simulink model "Appl_PaAdjustModel"  (R2018b)
settings: configuration reference "CodeConfig_10_ms" (kept outside this file)
undefined symbols (not defined in the file): CAL_HightMotorRunInterval_100ms, CAL_MotorDiffToStart_100ms, CAL_MotorStopTime_50ms, D_Relay_DownBackFault, D_Relay_UpFrontFault, D_ToleranceDistance, enSeatMoveCmd, FALSE, TRUE
libraries: DareLib x84, simulink x2
(part 1 of 3)
settings Model: Creator=Administrator  LastModifiedBy=Administrator
settings ConfigSetRef: SourceLocation=Base Workspace

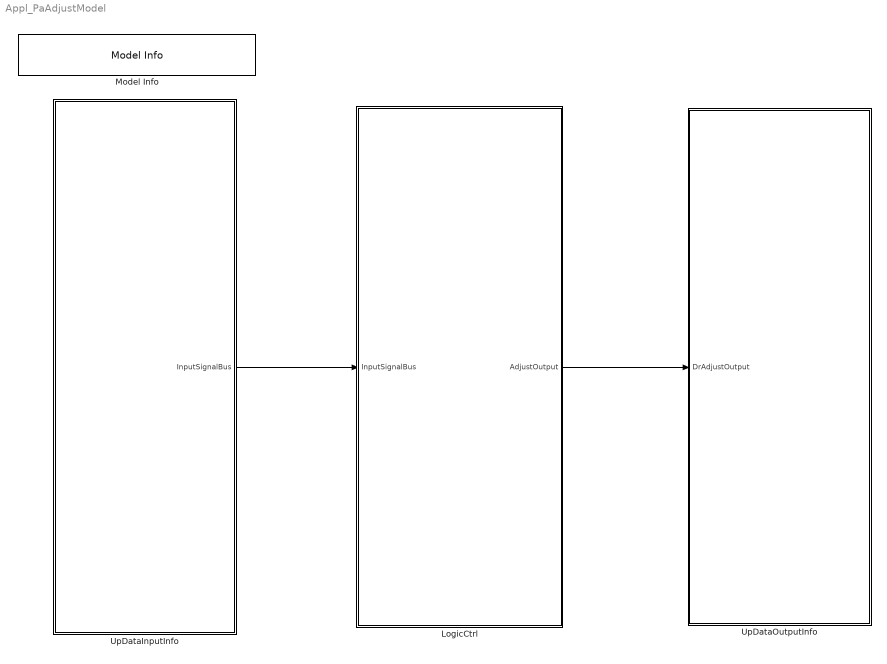
== system Appl_PaAdjustModel ==
  LogicCtrl : Subsystem  Priority=2  TreatAsAtomicUnit=on
      settings: RTWSystemCode=Nonreusable function  RTWFcnNameOpts=Use subsystem name
  Model Info : simulink/Model-Wide Utilities/Model Info  Frame=on  DisplayStringWithTags=Version：%<ModelVersion>  HorizontalTextAlignment=Center  LeftAlignmentValue=0.5
  UpDataInputInfo : Subsystem  Priority=1  TreatAsAtomicUnit=on
      settings: RTWSystemCode=Nonreusable function  RTWFcnNameOpts=Use subsystem name
  UpDataOutputInfo : Subsystem  Priority=3  TreatAsAtomicUnit=on
      settings: RTWSystemCode=Nonreusable function  RTWFcnNameOpts=Use subsystem name
  wires:
  UpDataInputInfo/1(InputSignalBus) -> LogicCtrl/1(InputSignalBus)
  LogicCtrl/1(AdjustOutput) -> UpDataOutputInfo/1(DrAdjustOutput)

== system Appl_PaAdjustModel/LogicCtrl ==
  InputSignalBus : Inport
  LocalAdjustCtrl : Subsystem  Description=调节逻辑处理
      settings: AttributesFormatString=%<Description>
  AdjustOutput : Outport
  wires:
  InputSignalBus/1 -> LocalAdjustCtrl/1(RteInputBus)  "RteInputBus"
  LocalAdjustCtrl/1(LocalAdjustCtrlOut) -> AdjustOutput/1

== system Appl_PaAdjustModel/UpDataInputInfo ==
  InputSignalProcess : Subsystem  Description=数据处理
      settings: AttributesFormatString=%<Description>  RTWSystemCode=Nonreusable function  RTWFcnNameOpts=Use subsystem name
  RTE : Subsystem  Description=接口自动生成  TreatAsAtomicUnit=on
      settings: AttributesFormatString=%<Description>  RTWSystemCode=Nonreusable function  RTWFcnNameOpts=Use subsystem name
  InputSignalBus : Outport
  wires:
  InputSignalProcess/1(InputSignalBus) -> InputSignalBus/1
  RTE/1(RTE_Signal) -> InputSignalProcess/1(Rte_SignalBus)

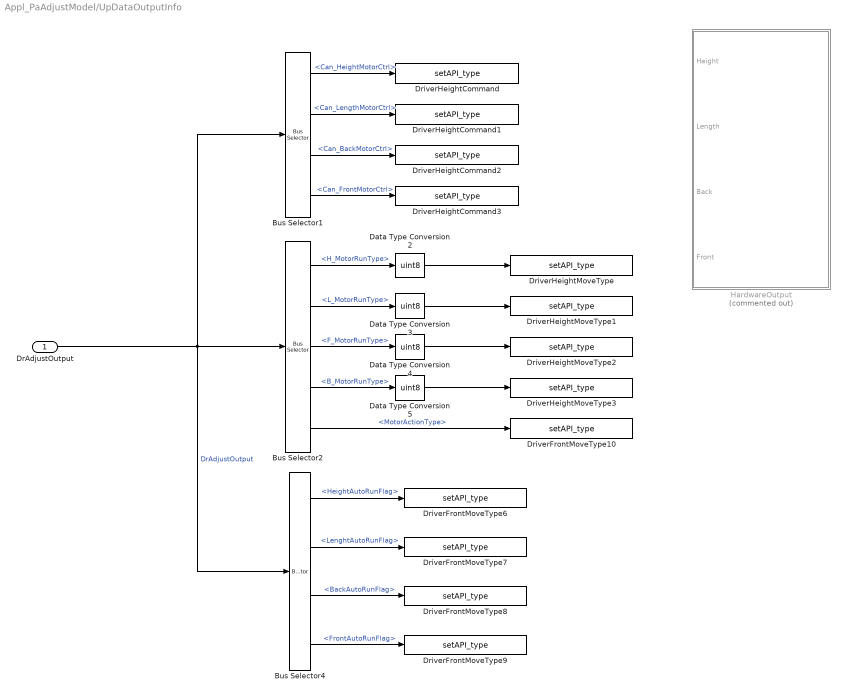
== system Appl_PaAdjustModel/UpDataOutputInfo ==
  DrAdjustOutput : Inport
  Bus Selector1 : BusSelector  OutputSignals=MotorCtrl.Can_HeightMotorCtrl,MotorCtrl.Can_LengthMotorCtrl,MotorCtrl.Can_BackMotorCtrl,MotorCtrl.Can_FrontMotorCtrl
  Bus Selector2 : BusSelector  OutputSignals=MotorRunType.H_MotorRunType,MotorRunType.L_MotorRunType,MotorRunType.F_MotorRunType,MotorRunType.B_MotorRunType,MotorReq.MotorActionType
  Bus Selector4 : BusSelector  OutputSignals=AutoRunFlag.HeightAutoRunFlag,AutoRunFlag.LenghtAutoRunFlag,AutoRunFlag.BackAutoRunFlag,AutoRunFlag.FrontAutoRunFlag
  Data Type Conversion{2..5} (4 alike) : DataTypeConversion  OutDataTypeStr=uint8
  DriverFrontMoveType10 : DareLib/Dare/setAPI_type  g_funcname=Rte_SetVfb_PaMoveType  g_param=""  g_type=uint8  g_enum=enSeatMotorRunTye  g_size=-1
      settings: AttributesFormatString=%<g_funcname>  SourceProductName=Dare Library
  DriverFrontMoveType6 : DareLib/Dare/setAPI_type  g_funcname=Rte_SetVfb_PaHeightAutoRunFlag  g_param=""  g_type=uint8  g_enum=enSeatAutoRunSts  g_size=-1
      settings: AttributesFormatString=%<g_funcname>  SourceProductName=Dare Library
  DriverFrontMoveType7 : DareLib/Dare/setAPI_type  g_funcname=Rte_SetVfb_PaLengthAutoRunFlag  g_param=""  g_type=uint8  g_enum=enSeatAutoRunSts  g_size=-1
      settings: AttributesFormatString=%<g_funcname>  SourceProductName=Dare Library
  DriverFrontMoveType8 : DareLib/Dare/setAPI_type  g_funcname=Rte_SetVfb_PaBackAutoRunFlag  g_param=""  g_type=uint8  g_enum=enSeatAutoRunSts  g_size=-1
      settings: AttributesFormatString=%<g_funcname>  SourceProductName=Dare Library
  DriverFrontMoveType9 : DareLib/Dare/setAPI_type  g_funcname=Rte_SetVfb_PaFrontAutoRunFlag  g_param=""  g_type=uint8  g_enum=enSeatAutoRunSts  g_size=-1
      settings: AttributesFormatString=%<g_funcname>  SourceProductName=Dare Library
  DriverHeightCommand : DareLib/Dare/setAPI_type  g_funcname=Rte_SetVfb_PaHeightMotorCmd  g_param=""  g_type=uint8  g_size=-1
      settings: AttributesFormatString=%<g_funcname>  SourceProductName=Dare Library
  DriverHeightCommand1 : DareLib/Dare/setAPI_type  g_funcname=Rte_SetVfb_PaLengthMotorCmd  g_param=""  g_type=uint8  g_size=-1
      settings: AttributesFormatString=%<g_funcname>  SourceProductName=Dare Library
  DriverHeightCommand2 : DareLib/Dare/setAPI_type  g_funcname=Rte_SetVfb_PaBackMotorCmd  g_param=""  g_type=uint8  g_size=-1
      settings: AttributesFormatString=%<g_funcname>  SourceProductName=Dare Library
  DriverHeightCommand3 : DareLib/Dare/setAPI_type  g_funcname=Rte_SetVfb_PaFrontMotorCmd  g_param=""  g_type=uint8  g_size=-1
      settings: AttributesFormatString=%<g_funcname>  SourceProductName=Dare Library
  DriverHeightMoveType : DareLib/Dare/setAPI_type  g_funcname=Rte_SetVfb_PaHeightMotorReason  g_param=""  g_type=uint8  g_size=-1
      settings: AttributesFormatString=%<g_funcname>  SourceProductName=Dare Library
  DriverHeightMoveType1 : DareLib/Dare/setAPI_type  g_funcname=Rte_SetVfb_PaLengthMotorReason  g_param=""  g_type=uint8  g_size=-1
      settings: AttributesFormatString=%<g_funcname>  SourceProductName=Dare Library
  DriverHeightMoveType2 : DareLib/Dare/setAPI_type  g_funcname=Rte_SetVfb_PaBackMotorReason  g_param=""  g_type=uint8  g_size=-1
      settings: AttributesFormatString=%<g_funcname>  SourceProductName=Dare Library
  DriverHeightMoveType3 : DareLib/Dare/setAPI_type  g_funcname=Rte_SetVfb_PaFrontMotorReason  g_param=""  g_type=uint8  g_size=-1
      settings: AttributesFormatString=%<g_funcname>  SourceProductName=Dare Library
  HardwareOutput : Subsystem  Commented=on
  wires:
  DrAdjustOutput/1 -> Bus Selector4/1, Bus Selector1/1, Bus Selector2/1  "DrAdjustOutput"
  Data Type Conversion2/1 -> DriverHeightMoveType/1
  Data Type Conversion3/1 -> DriverHeightMoveType1/1
  Data Type Conversion4/1 -> DriverHeightMoveType2/1
  Data Type Conversion5/1 -> DriverHeightMoveType3/1
  Bus Selector1/1 -> DriverHeightCommand/1  "<Can_HeightMotorCtrl>"
  Bus Selector1/2 -> DriverHeightCommand1/1  "<Can_LengthMotorCtrl>"
  Bus Selector1/3 -> DriverHeightCommand2/1  "<Can_BackMotorCtrl>"
  Bus Selector1/4 -> DriverHeightCommand3/1  "<Can_FrontMotorCtrl>"
  Bus Selector2/1 -> Data Type Conversion2/1  "<H_MotorRunType>"
  Bus Selector2/2 -> Data Type Conversion3/1  "<L_MotorRunType>"
  Bus Selector2/3 -> Data Type Conversion4/1  "<F_MotorRunType>"
  Bus Selector2/4 -> Data Type Conversion5/1  "<B_MotorRunType>"
  Bus Selector2/5 -> DriverFrontMoveType10/1  "<MotorActionType>"
  Bus Selector4/2 -> DriverFrontMoveType7/1  "<LenghtAutoRunFlag>"
  Bus Selector4/1 -> DriverFrontMoveType6/1  "<HeightAutoRunFlag>"
  Bus Selector4/3 -> DriverFrontMoveType8/1  "<BackAutoRunFlag>"
  Bus Selector4/4 -> DriverFrontMoveType9/1  "<FrontAutoRunFlag>"

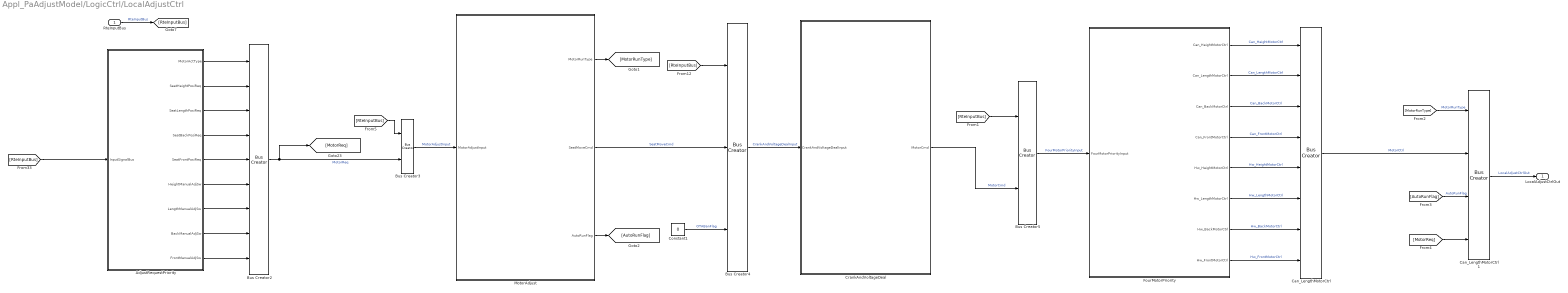
== system Appl_PaAdjustModel/LogicCtrl/LocalAdjustCtrl ==
  RteInputBus : Inport
  AdjustRequestPriority : Subsystem  Description=电机运动请求优先级处理
      settings: AttributesFormatString=%<Description>
      mask Display: image('优先级.png');
  Bus Creator2 : BusCreator  Inputs=9
  Bus Creator3 : BusCreator  Inputs=2
  Bus Creator4 : BusCreator  Inputs=3
  Bus Creator5 : BusCreator  Inputs=2
  Can_LengthMotorCtrl : BusCreator  Inputs=8
  Can_LengthMotorCtrl1 : BusCreator  Inputs=4
  Constant1 : Constant  Value=0
  CrankAndVoltageDeal : Subsystem  Description=CRANK卸荷和电压限制处理
      settings: AttributesFormatString=%<Description>
      mask Display: image('卸荷.png');
  FourMotorPriority : Subsystem  Description=四向调节电机运动优先级
      settings: AttributesFormatString=%<Description>
      mask Display: image('电机优先级.png');
  MotorAdjust : Subsystem  Description=四向电机调节
      settings: AttributesFormatString=%<Description>
      mask Display: image('电机调节.png');
  LocalAdjustCtrlOut : Outport
  wires:
  MotorAdjust/3(AutoRunFlag) -> [AutoRunFlag]
  [RteInputBus] -> Bus Creator4/1
  RteInputBus/1 -> [RteInputBus]  "RteInputBus"
  Bus Creator2/1 -> [MotorReq], Bus Creator3/2  "MotorReq"
  [RteInputBus] -> Bus Creator3/1
  Bus Creator3/1 -> MotorAdjust/1(MotorAdjustInput)  "MotorAdjustInput"
  Constant1/1 -> Bus Creator4/3  "OTABanFlag"
  MotorAdjust/2(SeatMoveCmd) -> Bus Creator4/2  "SeatMoveCmd"
  Bus Creator4/1 -> CrankAndVoltageDeal/1(CrankAndVoltageDealInput)  "CrankAndVoltageDealInput"
  CrankAndVoltageDeal/1(MotorCmd) -> Bus Creator5/2  "MotorCmd"
  [RteInputBus] -> Bus Creator5/1
  Bus Creator5/1 -> FourMotorPriority/1(FourMotorPriorityInput)  "FourMotorPriorityInput"
  MotorAdjust/1(MotorRunType) -> [MotorRunType]
  [MotorRunType] -> Can_LengthMotorCtrl1/1  "MotorRunType"
  [AutoRunFlag] -> Can_LengthMotorCtrl1/3  "AutoRunFlag"
  Can_LengthMotorCtrl/1 -> Can_LengthMotorCtrl1/2  "MotorCtrl"
  Can_LengthMotorCtrl1/1 -> LocalAdjustCtrlOut/1  "LocalAdjustCtrlOut"
  [MotorReq] -> Can_LengthMotorCtrl1/4
  AdjustRequestPriority/1(MotorActType) -> Bus Creator2/1
  AdjustRequestPriority/2(SeatHeightPosiReq) -> Bus Creator2/2
  AdjustRequestPriority/3(SeatLengthPosiReq) -> Bus Creator2/3
  AdjustRequestPriority/4(SeatBackPosiReq) -> Bus Creator2/4
  AdjustRequestPriority/5(SeatFrontPosiReq) -> Bus Creator2/5
  AdjustRequestPriority/6(HeightManualAdjSw) -> Bus Creator2/6
  AdjustRequestPriority/7(LengthManualAdjSw) -> Bus Creator2/7
  AdjustRequestPriority/8(BackManualAdjSw) -> Bus Creator2/8
  AdjustRequestPriority/9(FrontManualAdjSw) -> Bus Creator2/9
  FourMotorPriority/1(Can_HeightMotorCtrl) -> Can_LengthMotorCtrl/1  "Can_HeightMotorCtrl"
  FourMotorPriority/2(Can_LengthMotorCtrl) -> Can_LengthMotorCtrl/2  "Can_LengthMotorCtrl"
  FourMotorPriority/3(Can_BackMotorCtrl) -> Can_LengthMotorCtrl/3  "Can_BackMotorCtrl"
  FourMotorPriority/4(Can_FrontMotorCtrl) -> Can_LengthMotorCtrl/4  "Can_FrontMotorCtrl"
  FourMotorPriority/5(Hw_HeightMotorCtrl) -> Can_LengthMotorCtrl/5  "Hw_HeightMotorCtrl"
  FourMotorPriority/6(Hw_LengthMotorCtrl) -> Can_LengthMotorCtrl/6  "Hw_LengthMotorCtrl"
  FourMotorPriority/7(Hw_BackMotorCtrl) -> Can_LengthMotorCtrl/7  "Hw_BackMotorCtrl"
  FourMotorPriority/8(Hw_FrontMotorCtrl) -> Can_LengthMotorCtrl/8  "Hw_FrontMotorCtrl"
  [RteInputBus] -> AdjustRequestPriority/1(InputSignalBus)

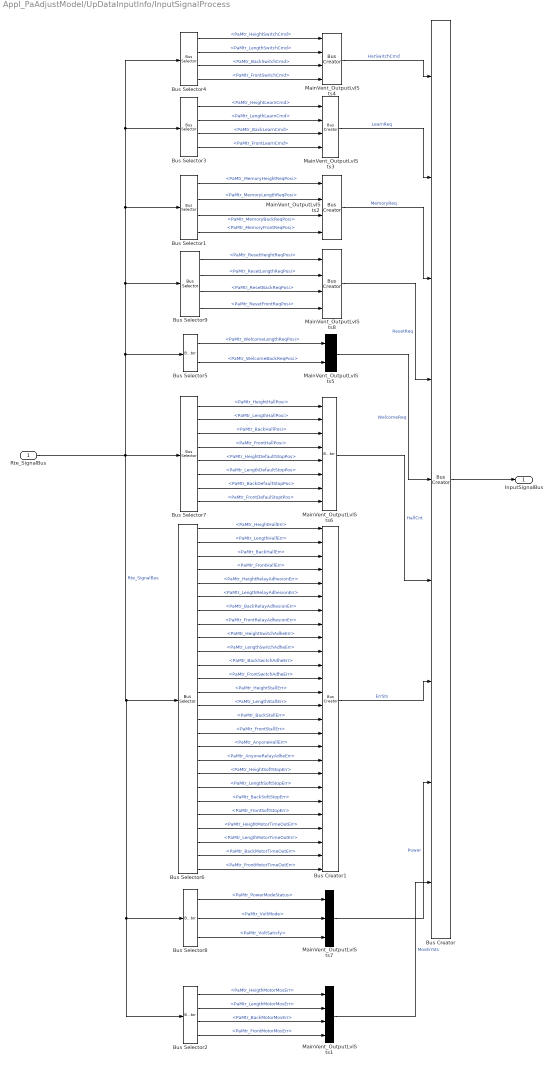
== system Appl_PaAdjustModel/UpDataInputInfo/InputSignalProcess ==
  Rte_SignalBus : Inport
  Bus Creator : BusCreator  Inputs=9
  Bus Creator1 : BusCreator  Inputs=26
  Bus Selector1 : BusSelector  OutputSignals=PaMtr_MemoryHeightReqPosi,PaMtr_MemoryLengthReqPosi,PaMtr_MemoryBackReqPosi,PaMtr_MemoryFrontReqPosi
  Bus Selector2 : BusSelector  OutputSignals=PaMtr_HeigthMotorMosErr,PaMtr_LengthMotorMosErr,PaMtr_BackMotorMosErr,PaMtr_FrontMotorMosErr
  Bus Selector3 : BusSelector  OutputSignals=PaMtr_HeightLearnCmd,PaMtr_LengthLearnCmd,PaMtr_BackLearnCmd,PaMtr_FrontLearnCmd
  Bus Selector4 : BusSelector  OutputSignals=PaMtr_HeightSwitchCmd,PaMtr_LengthSwitchCmd,PaMtr_BackSwitchCmd,PaMtr_FrontSwitchCmd
  Bus Selector5 : BusSelector  OutputSignals=PaMtr_WelcomeLengthReqPosi,PaMtr_WelcomeBackReqPosi
  Bus Selector6 : BusSelector  OutputSignals=PaMtr_HeightHallErr,PaMtr_LengthHallErr,PaMtr_BackHallErr,PaMtr_FrontHallErr,PaMtr_HeightRelayAdhesionErr,PaMtr_LengthRelayAdhesionErr,PaMtr_BackRelayAdhesionErr,PaMtr_FrontRelayAdhesionErr,PaMtr_HeightSwitchAdheErr,PaMtr_LengthSwitchAdheErr,PaMtr_BackSwitchAdheErr,PaMtr_FrontSwitchAdheErr,PaMtr_HeightStallErr,PaMtr_LengthStallErr,PaMtr_BackStallErr,PaMtr_FrontStallErr,PaMtr_AnyoneHallErr,PaMtr_AnyoneRelayAdheErr,PaMtr_HeightSoftStopErr,PaMtr_LengthSoftStopErr,PaMtr_BackSoftStopErr,PaMtr_FrontSoftStopErr,PaMtr_HeightMotorTimeOutErr,PaMtr_LengthMotorTimeOutErr,PaMtr_BackMotorTimeOutErr,PaMtr_FrontMotorTimeOutErr
  Bus Selector7 : BusSelector  OutputSignals=PaMtr_HeightHallPosi,PaMtr_LengthHallPosi,PaMtr_BackHallPosi,PaMtr_FrontHallPosi,PaMtr_HeightDefaultStopPos,PaMtr_LengthDefaultStopPos,PaMtr_BackDefaultStopPos,PaMtr_FrontDefaulStoptPos
  Bus Selector8 : BusSelector  OutputSignals=PaMtr_PowerModeStatus,PaMtr_VoltMode,PaMtr_VoltSatisfy
  Bus Selector9 : BusSelector  OutputSignals=PaMtr_ResetHeightReqPosi,PaMtr_ResetLengthReqPosi,PaMtr_ResetBackReqPosi,PaMtr_ResetFrontReqPosi
  MainVent_OutputLvlSts{1..4,8} (5 alike) : BusCreator  Inputs=4
  MainVent_OutputLvlSts5 : BusCreator  Inputs=2
  MainVent_OutputLvlSts6 : BusCreator  Inputs=8
  MainVent_OutputLvlSts7 : BusCreator  Inputs=3
  InputSignalBus : Outport
  wires:
  Bus Creator/1 -> InputSignalBus/1
  Bus Selector4/1 -> MainVent_OutputLvlSts4/1  "<PaMtr_HeightSwitchCmd>"
  Bus Selector4/2 -> MainVent_OutputLvlSts4/2  "<PaMtr_LengthSwitchCmd>"
  Bus Selector4/3 -> MainVent_OutputLvlSts4/3  "<PaMtr_BackSwitchCmd>"
  Bus Selector4/4 -> MainVent_OutputLvlSts4/4  "<PaMtr_FrontSwitchCmd>"
  Bus Selector7/1 -> MainVent_OutputLvlSts6/1  "<PaMtr_HeightHallPosi>"
  Bus Selector7/2 -> MainVent_OutputLvlSts6/2  "<PaMtr_LengthHallPosi>"
  Bus Selector7/3 -> MainVent_OutputLvlSts6/3  "<PaMtr_BackHallPosi>"
  Bus Selector7/4 -> MainVent_OutputLvlSts6/4  "<PaMtr_FrontHallPosi>"
  Bus Selector7/5 -> MainVent_OutputLvlSts6/5  "<PaMtr_HeightDefaultStopPos>"
  Bus Selector7/6 -> MainVent_OutputLvlSts6/6  "<PaMtr_LengthDefaultStopPos>"
  Bus Selector7/7 -> MainVent_OutputLvlSts6/7  "<PaMtr_BackDefaultStopPos>"
  Bus Selector8/2 -> MainVent_OutputLvlSts7/2  "<PaMtr_VoltMode>"
  Bus Selector8/1 -> MainVent_OutputLvlSts7/1  "<PaMtr_PowerModeStatus>"
  Bus Selector8/3 -> MainVent_OutputLvlSts7/3  "<PaMtr_VoltSatisfy>"
  MainVent_OutputLvlSts7/1 -> Bus Creator/8  "Power"
  MainVent_OutputLvlSts4/1 -> Bus Creator/1  "HarSwitchCmd"
  MainVent_OutputLvlSts2/1 -> Bus Creator/3  "MemoryReq"
  Bus Creator1/1 -> Bus Creator/7  "ErrSts"
  MainVent_OutputLvlSts5/1 -> Bus Creator/5  "WelcomeReq"
  MainVent_OutputLvlSts6/1 -> Bus Creator/6  "HallCnt"
  Bus Selector6/1 -> Bus Creator1/1  "<PaMtr_HeightHallErr>"
  Bus Selector6/2 -> Bus Creator1/2  "<PaMtr_LengthHallErr>"
  Bus Selector6/3 -> Bus Creator1/3  "<PaMtr_BackHallErr>"
  Bus Selector6/4 -> Bus Creator1/4  "<PaMtr_FrontHallErr>"
  Bus Selector6/5 -> Bus Creator1/5  "<PaMtr_HeightRelayAdhesionErr>"
  Bus Selector6/6 -> Bus Creator1/6  "<PaMtr_LengthRelayAdhesionErr>"
  Bus Selector6/7 -> Bus Creator1/7  "<PaMtr_BackRelayAdhesionErr>"
  Bus Selector6/8 -> Bus Creator1/8  "<PaMtr_FrontRelayAdhesionErr>"
  Bus Selector6/9 -> Bus Creator1/9  "<PaMtr_HeightSwitchAdheErr>"
  Bus Selector6/10 -> Bus Creator1/10  "<PaMtr_LengthSwitchAdheErr>"
  Bus Selector6/11 -> Bus Creator1/11  "<PaMtr_BackSwitchAdheErr>"
  Bus Selector6/12 -> Bus Creator1/12  "<PaMtr_FrontSwitchAdheErr>"
  Bus Selector6/13 -> Bus Creator1/13  "<PaMtr_HeightStallErr>"
  Bus Selector6/14 -> Bus Creator1/14  "<PaMtr_LengthStallErr>"
  Bus Selector6/15 -> Bus Creator1/15  "<PaMtr_BackStallErr>"
  Bus Selector6/16 -> Bus Creator1/16  "<PaMtr_FrontStallErr>"
  Bus Selector6/17 -> Bus Creator1/17  "<PaMtr_AnyoneHallErr>"
  Bus Selector6/18 -> Bus Creator1/18  "<PaMtr_AnyoneRelayAdheErr>"
  Bus Selector6/19 -> Bus Creator1/19  "<PaMtr_HeightSoftStopErr>"
  Bus Selector6/20 -> Bus Creator1/20  "<PaMtr_LengthSoftStopErr>"
  Bus Selector6/21 -> Bus Creator1/21  "<PaMtr_BackSoftStopErr>"
  Bus Selector6/22 -> Bus Creator1/22  "<PaMtr_FrontSoftStopErr>"
  Bus Selector6/23 -> Bus Creator1/23  "<PaMtr_HeightMotorTimeOutErr>"
  Bus Selector6/24 -> Bus Creator1/24  "<PaMtr_LengthMotorTimeOutErr>"
  Bus Selector6/25 -> Bus Creator1/25  "<PaMtr_BackMotorTimeOutErr>"
  Bus Selector6/26 -> Bus Creator1/26  "<PaMtr_FrontMotorTimeOutErr>"
  Bus Selector1/3 -> MainVent_OutputLvlSts2/3  "<PaMtr_MemoryBackReqPosi>"
  Bus Selector1/2 -> MainVent_OutputLvlSts2/2  "<PaMtr_MemoryLengthReqPosi>"
  Bus Selector1/4 -> MainVent_OutputLvlSts2/4  "<PaMtr_MemoryFrontReqPosi>"
  Bus Selector1/1 -> MainVent_OutputLvlSts2/1  "<PaMtr_MemoryHeightReqPosi>"
  Bus Selector5/1 -> MainVent_OutputLvlSts5/1  "<PaMtr_WelcomeLengthReqPosi>"
  Bus Selector5/2 -> MainVent_OutputLvlSts5/2  "<PaMtr_WelcomeBackReqPosi>"
  Bus Selector7/8 -> MainVent_OutputLvlSts6/8  "<PaMtr_FrontDefaulStoptPos>"
  Bus Selector3/1 -> MainVent_OutputLvlSts3/1  "<PaMtr_HeightLearnCmd>"
  Bus Selector3/2 -> MainVent_OutputLvlSts3/2  "<PaMtr_LengthLearnCmd>"
  Bus Selector3/3 -> MainVent_OutputLvlSts3/3  "<PaMtr_BackLearnCmd>"
  Bus Selector3/4 -> MainVent_OutputLvlSts3/4  "<PaMtr_FrontLearnCmd>"
  MainVent_OutputLvlSts3/1 -> Bus Creator/2  "LearnReq"
  Bus Selector9/1 -> MainVent_OutputLvlSts8/1  "<PaMtr_ResetHeightReqPosi>"
  Bus Selector9/2 -> MainVent_OutputLvlSts8/2  "<PaMtr_ResetLengthReqPosi>"
  Bus Selector9/4 -> MainVent_OutputLvlSts8/4  "<PaMtr_ResetFrontReqPosi>"
  Bus Selector9/3 -> MainVent_OutputLvlSts8/3  "<PaMtr_ResetBackReqPosi>"
  MainVent_OutputLvlSts8/1 -> Bus Creator/4  "ResetReq"
  MainVent_OutputLvlSts1/1 -> Bus Creator/9  "MosErrSts"
  Bus Selector2/3 -> MainVent_OutputLvlSts1/3  "<PaMtr_BackMotorMosErr>"
  Bus Selector2/2 -> MainVent_OutputLvlSts1/2  "<PaMtr_LengthMotorMosErr>"
  Rte_SignalBus/1 -> Bus Selector2/1, Bus Selector8/1, Bus Selector6/1, Bus Selector7/1, Bus Selector4/1, Bus Selector3/1, Bus Selector1/1, Bus Selector9/1, Bus Selector5/1  "Rte_SignalBus"
  Bus Selector2/4 -> MainVent_OutputLvlSts1/4  "<PaMtr_FrontMotorMosErr>"
  Bus Selector2/1 -> MainVent_OutputLvlSts1/1  "<PaMtr_HeigthMotorMosErr>"

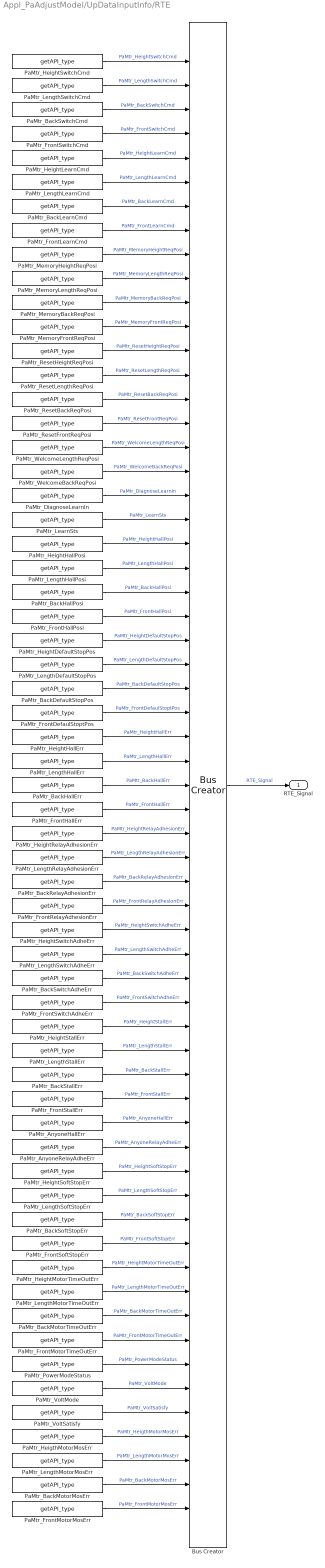
== system Appl_PaAdjustModel/UpDataInputInfo/RTE ==
  Bus Creator : BusCreator  Inputs=61
  PaMtr_AnyoneHallErr : DareLib/Dare/getAPI_type  g_funcname=Rte_GetVfb_PaAnyoneHallErr  g_param=""  g_type=uint8  g_size=-1
      settings: AttributesFormatString=%<g_funcname>  SourceProductName=Dare Library
  PaMtr_AnyoneRelayAdheErr : DareLib/Dare/getAPI_type  g_funcname=Rte_GetVfb_PaAnyoneRelayAdheErr  g_param=""  g_type=uint8  g_size=-1
      settings: AttributesFormatString=%<g_funcname>  SourceProductName=Dare Library
  PaMtr_BackDefaultStopPos : DareLib/Dare/getAPI_type  g_funcname=Cdd_GetMotorHardStop  g_param=EN_PassengerBack  g_type=uint16  g_size=-1
      settings: AttributesFormatString=%<g_funcname>  SourceProductName=Dare Library
  PaMtr_BackHallErr : DareLib/Dare/getAPI_type  g_funcname=Rte_GetVfb_PaBackHallErr  g_param=""  g_type=uint8  g_size=-1
      settings: AttributesFormatString=%<g_funcname>  SourceProductName=Dare Library
  PaMtr_BackHallPosi : DareLib/Dare/getAPI_type  g_funcname=Cdd_GetCurrentHallCnt  g_param=EN_PassengerBack  g_type=uint16  g_size=-1
      settings: AttributesFormatString=%<g_funcname>  SourceProductName=Dare Library
  PaMtr_BackLearnCmd : DareLib/Dare/getAPI_type  g_funcname=Rte_GetVfb_PaBackLearnCmd  g_param=""  g_type=uint8  g_size=-1
      settings: AttributesFormatString=%<g_funcname>  SourceProductName=Dare Library
  PaMtr_BackMotorMosErr : DareLib/Dare/getAPI_type  g_funcname=Srvl_Tle9210x_GetMotorErr  g_param=EN_SEAT_PAS_BACK  g_type=uint8  g_enum=enMosErrSts  g_size=-1
      settings: AttributesFormatString=%<g_funcname>  SourceProductName=Dare Library
  PaMtr_BackMotorTimeOutErr : DareLib/Dare/getAPI_type  g_funcname=Rte_GetVfb_PaBackMotorTimeOutErr  g_param=""  g_type=uint8  g_size=-1
      settings: AttributesFormatString=%<g_funcname>  SourceProductName=Dare Library
  PaMtr_BackRelayAdhesionErr : DareLib/Dare/getAPI_type  g_funcname=Rte_GetVfb_PaBackRelayAdheErr  g_param=""  g_type=uint8  g_size=-1
      settings: AttributesFormatString=%<g_funcname>  SourceProductName=Dare Library
  PaMtr_BackSoftStopErr : DareLib/Dare/getAPI_type  g_funcname=Rte_GetVfb_PaBackSoftStopErr  g_param=""  g_type=uint8  g_size=-1
      settings: AttributesFormatString=%<g_funcname>  SourceProductName=Dare Library
  PaMtr_BackStallErr : DareLib/Dare/getAPI_type  g_funcname=Rte_GetVfb_PaBackStallErr  g_param=""  g_type=uint8  g_size=-1
      settings: AttributesFormatString=%<g_funcname>  SourceProductName=Dare Library
  PaMtr_BackSwitchAdheErr : DareLib/Dare/getAPI_type  g_funcname=Rte_GetVfb_PaBackSwitchAdheErr  g_param=""  g_type=uint8  g_size=-1
      settings: AttributesFormatString=%<g_funcname>  SourceProductName=Dare Library
  PaMtr_BackSwitchCmd : DareLib/Dare/getAPI_type  g_funcname=Rte_GetVfb_PaBackSwitchCmd  g_param=""  g_type=uint8  g_size=-1
      settings: AttributesFormatString=%<g_funcname>  SourceProductName=Dare Library
  PaMtr_DiagnoseLearnIn : DareLib/Dare/getAPI_type  g_funcname=Rte_GetVfb_PaLearnEnable  g_param=""  g_type=uint8  g_size=-1
      settings: AttributesFormatString=%<g_funcname>  SourceProductName=Dare Library
  PaMtr_FrontDefaulStoptPos : DareLib/Dare/getAPI_type  g_funcname=Cdd_GetMotorHardStop  g_param=EN_PaResever_2  g_type=uint16  g_size=-1
      settings: AttributesFormatString=%<g_funcname>  SourceProductName=Dare Library
  PaMtr_FrontHallErr : DareLib/Dare/getAPI_type  g_funcname=Rte_GetVfb_PaFrontHallErr  g_param=""  g_type=uint8  g_size=-1
      settings: AttributesFormatString=%<g_funcname>  SourceProductName=Dare Library
  PaMtr_FrontHallPosi : DareLib/Dare/getAPI_type  g_funcname=Cdd_GetCurrentHallCnt  g_param=EN_PaResever_2  g_type=uint16  g_size=-1
      settings: AttributesFormatString=%<g_funcname>  SourceProductName=Dare Library
  PaMtr_FrontLearnCmd : DareLib/Dare/getAPI_type  g_funcname=Rte_GetVfb_PaFrontLearnCmd  g_param=""  g_type=uint8  g_size=-1
      settings: AttributesFormatString=%<g_funcname>  SourceProductName=Dare Library
  PaMtr_FrontMotorMosErr : DareLib/Dare/getAPI_type  g_funcname=Srvl_Tle9210x_GetMotorErr  g_param=EN_SEAT_PAS_FRONT  g_type=uint8  g_enum=enMosErrSts  g_size=-1
      settings: AttributesFormatString=%<g_funcname>  SourceProductName=Dare Library
  PaMtr_FrontMotorTimeOutErr : DareLib/Dare/getAPI_type  g_funcname=Rte_GetVfb_PaFrontMotorTimeOutErr  g_param=""  g_type=uint8  g_size=-1
      settings: AttributesFormatString=%<g_funcname>  SourceProductName=Dare Library
  PaMtr_FrontRelayAdhesionErr : DareLib/Dare/getAPI_type  g_funcname=Rte_GetVfb_PaFrontRelayAdheErr  g_param=""  g_type=uint8  g_size=-1
      settings: AttributesFormatString=%<g_funcname>  SourceProductName=Dare Library
  PaMtr_FrontSoftStopErr : DareLib/Dare/getAPI_type  g_funcname=Rte_GetVfb_PaFrontSoftStopErr  g_param=""  g_type=uint8  g_size=-1
      settings: AttributesFormatString=%<g_funcname>  SourceProductName=Dare Library
  PaMtr_FrontStallErr : DareLib/Dare/getAPI_type  g_funcname=Rte_GetVfb_PaFrontStallErr  g_param=""  g_type=uint8  g_size=-1
      settings: AttributesFormatString=%<g_funcname>  SourceProductName=Dare Library
  PaMtr_FrontSwitchAdheErr : DareLib/Dare/getAPI_type  g_funcname=Rte_GetVfb_PaFrontSwitchAdheErr  g_param=""  g_type=uint8  g_size=-1
      settings: AttributesFormatString=%<g_funcname>  SourceProductName=Dare Library
  PaMtr_FrontSwitchCmd : DareLib/Dare/getAPI_type  g_funcname=Rte_GetVfb_PaFrontSwitchCmd  g_param=""  g_type=uint8  g_size=-1
      settings: AttributesFormatString=%<g_funcname>  SourceProductName=Dare Library
  PaMtr_HeightDefaultStopPos : DareLib/Dare/getAPI_type  g_funcname=Cdd_GetMotorHardStop  g_param=EN_PaResever_1  g_type=uint16  g_size=-1
      settings: AttributesFormatString=%<g_funcname>  SourceProductName=Dare Library
  PaMtr_HeightHallErr : DareLib/Dare/getAPI_type  g_funcname=Rte_GetVfb_PaHeightHallErr  g_param=""  g_type=uint8  g_size=-1
      settings: AttributesFormatString=%<g_funcname>  SourceProductName=Dare Library
  PaMtr_HeightHallPosi : DareLib/Dare/getAPI_type  g_funcname=Cdd_GetCurrentHallCnt  g_param=EN_PaResever_1  g_type=uint16  g_size=-1
      settings: AttributesFormatString=%<g_funcname>  SourceProductName=Dare Library
  PaMtr_HeightLearnCmd : DareLib/Dare/getAPI_type  g_funcname=Rte_GetVfb_PaHeightLearnCmd  g_param=""  g_type=uint8  g_size=-1
      settings: AttributesFormatString=%<g_funcname>  SourceProductName=Dare Library
  PaMtr_HeightMotorTimeOutErr : DareLib/Dare/getAPI_type  g_funcname=Rte_GetVfb_PaHeightMotorTimeOutErr  g_param=""  g_type=uint8  g_size=-1
      settings: AttributesFormatString=%<g_funcname>  SourceProductName=Dare Library
  PaMtr_HeightRelayAdhesionErr : DareLib/Dare/getAPI_type  g_funcname=Rte_GetVfb_PaHeightRelayAdheErr  g_param=""  g_type=uint8  g_size=-1
      settings: AttributesFormatString=%<g_funcname>  SourceProductName=Dare Library
  PaMtr_HeightSoftStopErr : DareLib/Dare/getAPI_type  g_funcname=Rte_GetVfb_PaLengthSoftStopErr  g_param=""  g_type=uint8  g_size=-1
      settings: AttributesFormatString=%<g_funcname>  SourceProductName=Dare Library
  PaMtr_HeightStallErr : DareLib/Dare/getAPI_type  g_funcname=Rte_GetVfb_PaHeightStallErr  g_param=""  g_type=uint8  g_size=-1
      settings: AttributesFormatString=%<g_funcname>  SourceProductName=Dare Library
  PaMtr_HeightSwitchAdheErr : DareLib/Dare/getAPI_type  g_funcname=Rte_GetVfb_PaHeightSwitchAdheErr  g_param=""  g_type=uint8  g_size=-1
      settings: AttributesFormatString=%<g_funcname>  SourceProductName=Dare Library
  PaMtr_HeightSwitchCmd : DareLib/Dare/getAPI_type  g_funcname=Rte_GetVfb_PaHeightSwitchCmd  g_param=""  g_type=uint8  g_size=-1
      settings: AttributesFormatString=%<g_funcname>  SourceProductName=Dare Library
  PaMtr_HeigthMotorMosErr : DareLib/Dare/getAPI_type  g_funcname=Srvl_Tle9210x_GetMotorErr  g_param=EN_SEAT_PAS_HEIGHT  g_type=uint8  g_enum=enMosErrSts  g_size=-1
      settings: AttributesFormatString=%<g_funcname>  SourceProductName=Dare Library
  PaMtr_LearnSts : DareLib/Dare/getAPI_type  g_funcname=Rte_GetVfb_PaLearnSts  g_param=""  g_type=uint8  g_size=-1
      settings: AttributesFormatString=%<g_funcname>  SourceProductName=Dare Library
  PaMtr_LengthDefaultStopPos : DareLib/Dare/getAPI_type  g_funcname=Cdd_GetMotorHardStop  g_param=EN_PassengerLength  g_type=uint16  g_size=-1
      settings: AttributesFormatString=%<g_funcname>  SourceProductName=Dare Library
  PaMtr_LengthHallErr : DareLib/Dare/getAPI_type  g_funcname=Rte_GetVfb_PaLengthHallErr  g_param=""  g_type=uint8  g_size=-1
      settings: AttributesFormatString=%<g_funcname>  SourceProductName=Dare Library
  PaMtr_LengthHallPosi : DareLib/Dare/getAPI_type  g_funcname=Cdd_GetCurrentHallCnt  g_param=EN_PassengerLength  g_type=uint16  g_size=-1
      settings: AttributesFormatString=%<g_funcname>  SourceProductName=Dare Library
  PaMtr_LengthLearnCmd : DareLib/Dare/getAPI_type  g_funcname=Rte_GetVfb_PaLengthLearnCmd  g_param=""  g_type=uint8  g_size=-1
      settings: AttributesFormatString=%<g_funcname>  SourceProductName=Dare Library
  PaMtr_LengthMotorMosErr : DareLib/Dare/getAPI_type  g_funcname=Srvl_Tle9210x_GetMotorErr  g_param=EN_SEAT_PAS_LENGTH  g_type=uint8  g_enum=enMosErrSts  g_size=-1
      settings: AttributesFormatString=%<g_funcname>  SourceProductName=Dare Library
  PaMtr_LengthMotorTimeOutErr : DareLib/Dare/getAPI_type  g_funcname=Rte_GetVfb_PaLengthMotorTimeOutErr  g_param=""  g_type=uint8  g_size=-1
      settings: AttributesFormatString=%<g_funcname>  SourceProductName=Dare Library
  PaMtr_LengthRelayAdhesionErr : DareLib/Dare/getAPI_type  g_funcname=Rte_GetVfb_PaLengthRelayAdheErr  g_param=""  g_type=uint8  g_size=-1
      settings: AttributesFormatString=%<g_funcname>  SourceProductName=Dare Library
  PaMtr_LengthSoftStopErr : DareLib/Dare/getAPI_type  g_funcname=Rte_GetVfb_PaHeightSoftStopErr  g_param=""  g_type=uint8  g_size=-1
      settings: AttributesFormatString=%<g_funcname>  SourceProductName=Dare Library
  PaMtr_LengthStallErr : DareLib/Dare/getAPI_type  g_funcname=Rte_GetVfb_PaLengthStallErr  g_param=""  g_type=uint8  g_size=-1
      settings: AttributesFormatString=%<g_funcname>  SourceProductName=Dare Library
  PaMtr_LengthSwitchAdheErr : DareLib/Dare/getAPI_type  g_funcname=Rte_GetVfb_PaLengthSwitchAdheErr  g_param=""  g_type=uint8  g_size=-1
      settings: AttributesFormatString=%<g_funcname>  SourceProductName=Dare Library
  PaMtr_LengthSwitchCmd : DareLib/Dare/getAPI_type  g_funcname=Rte_GetVfb_PaLengthSwitchCmd  g_param=""  g_type=uint8  g_size=-1
      settings: AttributesFormatString=%<g_funcname>  SourceProductName=Dare Library
  PaMtr_MemoryBackReqPosi : DareLib/Dare/getAPI_type  g_funcname=Rte_GetVfb_PaMemBackReqPosi  g_param=""  g_type=uint16  g_size=-1
      settings: AttributesFormatString=%<g_funcname>  SourceProductName=Dare Library
  PaMtr_MemoryFrontReqPosi : DareLib/Dare/getAPI_type  g_funcname=Rte_GetVfb_PaMemFrontReqPosi  g_param=""  g_type=uint16  g_size=-1
      settings: AttributesFormatString=%<g_funcname>  SourceProductName=Dare Library
  PaMtr_MemoryHeightReqPosi : DareLib/Dare/getAPI_type  g_funcname=Rte_GetVfb_PaMemHeightReqPosi  g_param=""  g_type=uint16  g_size=-1
      settings: AttributesFormatString=%<g_funcname>  SourceProductName=Dare Library
  PaMtr_MemoryLengthReqPosi : DareLib/Dare/getAPI_type  g_funcname=Rte_GetVfb_PaMemLengthReqPosi  g_param=""  g_type=uint16  g_size=-1
      settings: AttributesFormatString=%<g_funcname>  SourceProductName=Dare Library
  PaMtr_PowerModeStatus : DareLib/Dare/getAPI_type  g_funcname=Rte_GetVfb_PowerMode  g_param=""  g_type=uint8  g_enum=enIgnSts  g_size=-1
      settings: AttributesFormatString=%<g_funcname>  SourceProductName=Dare Library
  PaMtr_ResetBackReqPosi : DareLib/Dare/getAPI_type  g_funcname=Rte_GetVfb_PaBackResetReqPosi  g_param=""  g_type=uint16  g_size=-1
      settings: AttributesFormatString=%<g_funcname>  SourceProductName=Dare Library
  PaMtr_ResetFrontReqPosi : DareLib/Dare/getAPI_type  g_funcname=Rte_GetVfb_PaFrontResetReqPosi  g_param=""  g_type=uint16  g_size=-1
      settings: AttributesFormatString=%<g_funcname>  SourceProductName=Dare Library
  PaMtr_ResetHeightReqPosi : DareLib/Dare/getAPI_type  g_funcname=Rte_GetVfb_PaHeightResetReqPosi  g_param=""  g_type=uint16  g_size=-1
      settings: AttributesFormatString=%<g_funcname>  SourceProductName=Dare Library
  PaMtr_ResetLengthReqPosi : DareLib/Dare/getAPI_type  g_funcname=Rte_GetVfb_PaLengthResetReqPosi  g_param=""  g_type=uint16  g_size=-1
      settings: AttributesFormatString=%<g_funcname>  SourceProductName=Dare Library
  PaMtr_VoltMode : DareLib/Dare/getAPI_type  g_funcname=Rte_GetVfb_VoltMode  g_param=""  g_type=uint8  g_enum=enFinalPowerMode  g_size=-1
      settings: AttributesFormatString=%<g_funcname>  SourceProductName=Dare Library
  PaMtr_VoltSatisfy : DareLib/Dare/getAPI_type  g_funcname=Rte_GetVfb_VoltSatisfy  g_param=""  g_type=uint8  g_size=-1
      settings: AttributesFormatString=%<g_funcname>  SourceProductName=Dare Library
  PaMtr_WelcomeBackReqPosi : DareLib/Dare/getAPI_type  g_funcname=Rte_GetVfb_PaWelBackReqPosi  g_param=""  g_type=uint16  g_size=-1
      settings: AttributesFormatString=%<g_funcname>  SourceProductName=Dare Library
  PaMtr_WelcomeLengthReqPosi : DareLib/Dare/getAPI_type  g_funcname=Rte_GetVfb_PaWelLengthReqPosi  g_param=""  g_type=uint16  g_size=-1
      settings: AttributesFormatString=%<g_funcname>  SourceProductName=Dare Library
  RTE_Signal : Outport
  wires:
  Bus Creator/1 -> RTE_Signal/1  "RTE_Signal"
  PaMtr_ResetHeightReqPosi/1 -> Bus Creator/13  "PaMtr_ResetHeightReqPosi"
  PaMtr_MemoryFrontReqPosi/1 -> Bus Creator/12  "PaMtr_MemoryFrontReqPosi"
  PaMtr_ResetLengthReqPosi/1 -> Bus Creator/14  "PaMtr_ResetLengthReqPosi"
  PaMtr_MemoryBackReqPosi/1 -> Bus Creator/11  "PaMtr_MemoryBackReqPosi"
  PaMtr_ResetBackReqPosi/1 -> Bus Creator/15  "PaMtr_ResetBackReqPosi"
  PaMtr_MemoryLengthReqPosi/1 -> Bus Creator/10  "PaMtr_MemoryLengthReqPosi"
  PaMtr_ResetFrontReqPosi/1 -> Bus Creator/16  "PaMtr_ResetFrontReqPosi"
  PaMtr_MemoryHeightReqPosi/1 -> Bus Creator/9  "PaMtr_MemoryHeightReqPosi"
  PaMtr_WelcomeLengthReqPosi/1 -> Bus Creator/17  "PaMtr_WelcomeLengthReqPosi"
  PaMtr_FrontLearnCmd/1 -> Bus Creator/8  "PaMtr_FrontLearnCmd"
  PaMtr_WelcomeBackReqPosi/1 -> Bus Creator/18  "PaMtr_WelcomeBackReqPosi"
  PaMtr_BackLearnCmd/1 -> Bus Creator/7  "PaMtr_BackLearnCmd"
  PaMtr_DiagnoseLearnIn/1 -> Bus Creator/19  "PaMtr_DiagnoseLearnIn"
  PaMtr_LengthLearnCmd/1 -> Bus Creator/6  "PaMtr_LengthLearnCmd"
  PaMtr_LearnSts/1 -> Bus Creator/20  "PaMtr_LearnSts"
  PaMtr_HeightLearnCmd/1 -> Bus Creator/5  "PaMtr_HeightLearnCmd"
  PaMtr_HeightHallPosi/1 -> Bus Creator/21  "PaMtr_HeightHallPosi"
  PaMtr_FrontSwitchCmd/1 -> Bus Creator/4  "PaMtr_FrontSwitchCmd"
  PaMtr_LengthHallPosi/1 -> Bus Creator/22  "PaMtr_LengthHallPosi"
  PaMtr_BackSwitchCmd/1 -> Bus Creator/3  "PaMtr_BackSwitchCmd"
  PaMtr_BackHallPosi/1 -> Bus Creator/23  "PaMtr_BackHallPosi"
  PaMtr_LengthSwitchCmd/1 -> Bus Creator/2  "PaMtr_LengthSwitchCmd"
  PaMtr_FrontHallPosi/1 -> Bus Creator/24  "PaMtr_FrontHallPosi"
  PaMtr_HeightSwitchCmd/1 -> Bus Creator/1  "PaMtr_HeightSwitchCmd"
  PaMtr_HeightDefaultStopPos/1 -> Bus Creator/25  "PaMtr_HeightDefaultStopPos"
  PaMtr_LengthDefaultStopPos/1 -> Bus Creator/26  "PaMtr_LengthDefaultStopPos"
  PaMtr_BackDefaultStopPos/1 -> Bus Creator/27  "PaMtr_BackDefaultStopPos"
  PaMtr_FrontDefaulStoptPos/1 -> Bus Creator/28  "PaMtr_FrontDefaulStoptPos"
  PaMtr_HeightHallErr/1 -> Bus Creator/29  "PaMtr_HeightHallErr"
  PaMtr_LengthHallErr/1 -> Bus Creator/30  "PaMtr_LengthHallErr"
  PaMtr_BackHallErr/1 -> Bus Creator/31  "PaMtr_BackHallErr"
  PaMtr_FrontHallErr/1 -> Bus Creator/32  "PaMtr_FrontHallErr"
  PaMtr_HeightRelayAdhesionErr/1 -> Bus Creator/33  "PaMtr_HeightRelayAdhesionErr"
  PaMtr_LengthRelayAdhesionErr/1 -> Bus Creator/34  "PaMtr_LengthRelayAdhesionErr"
  PaMtr_BackRelayAdhesionErr/1 -> Bus Creator/35  "PaMtr_BackRelayAdhesionErr"
  PaMtr_FrontRelayAdhesionErr/1 -> Bus Creator/36  "PaMtr_FrontRelayAdhesionErr"
  PaMtr_HeightSwitchAdheErr/1 -> Bus Creator/37  "PaMtr_HeightSwitchAdheErr"
  PaMtr_LengthSwitchAdheErr/1 -> Bus Creator/38  "PaMtr_LengthSwitchAdheErr"
  PaMtr_BackSwitchAdheErr/1 -> Bus Creator/39  "PaMtr_BackSwitchAdheErr"
  PaMtr_FrontSwitchAdheErr/1 -> Bus Creator/40  "PaMtr_FrontSwitchAdheErr"
  PaMtr_HeightStallErr/1 -> Bus Creator/41  "PaMtr_HeightStallErr"
  PaMtr_LengthStallErr/1 -> Bus Creator/42  "PaMtr_LengthStallErr"
  PaMtr_BackStallErr/1 -> Bus Creator/43  "PaMtr_BackStallErr"
  PaMtr_FrontStallErr/1 -> Bus Creator/44  "PaMtr_FrontStallErr"
  PaMtr_AnyoneHallErr/1 -> Bus Creator/45  "PaMtr_AnyoneHallErr"
  PaMtr_AnyoneRelayAdheErr/1 -> Bus Creator/46  "PaMtr_AnyoneRelayAdheErr"
  PaMtr_HeightSoftStopErr/1 -> Bus Creator/47  "PaMtr_HeightSoftStopErr"
  PaMtr_LengthSoftStopErr/1 -> Bus Creator/48  "PaMtr_LengthSoftStopErr"
  PaMtr_BackSoftStopErr/1 -> Bus Creator/49  "PaMtr_BackSoftStopErr"
  PaMtr_FrontSoftStopErr/1 -> Bus Creator/50  "PaMtr_FrontSoftStopErr"
  PaMtr_HeightMotorTimeOutErr/1 -> Bus Creator/51  "PaMtr_HeightMotorTimeOutErr"
  PaMtr_LengthMotorTimeOutErr/1 -> Bus Creator/52  "PaMtr_LengthMotorTimeOutErr"
  PaMtr_BackMotorTimeOutErr/1 -> Bus Creator/53  "PaMtr_BackMotorTimeOutErr"
  PaMtr_FrontMotorTimeOutErr/1 -> Bus Creator/54  "PaMtr_FrontMotorTimeOutErr"
  PaMtr_PowerModeStatus/1 -> Bus Creator/55  "PaMtr_PowerModeStatus"
  PaMtr_VoltMode/1 -> Bus Creator/56  "PaMtr_VoltMode"
  PaMtr_VoltSatisfy/1 -> Bus Creator/57  "PaMtr_VoltSatisfy"
  PaMtr_HeigthMotorMosErr/1 -> Bus Creator/58  "PaMtr_HeigthMotorMosErr"
  PaMtr_LengthMotorMosErr/1 -> Bus Creator/59  "PaMtr_LengthMotorMosErr"
  PaMtr_BackMotorMosErr/1 -> Bus Creator/60  "PaMtr_BackMotorMosErr"
  PaMtr_FrontMotorMosErr/1 -> Bus Creator/61  "PaMtr_FrontMotorMosErr"

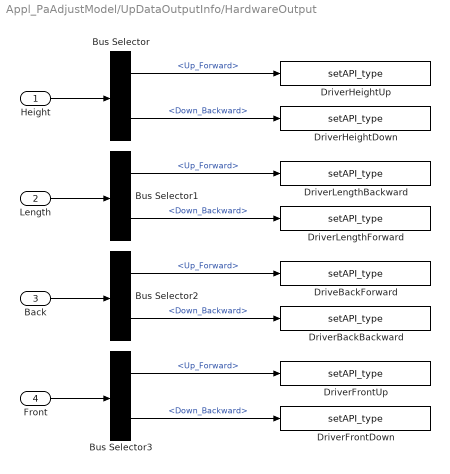
== system Appl_PaAdjustModel/UpDataOutputInfo/HardwareOutput ==
  Height : Inport
  Length : Inport  Port=2
  Back : Inport  Port=3
  Front : Inport  Port=4
  Bus Selector{,1..3} (4 alike) : BusSelector  OutputSignals=Up_Forward,Down_Backward
  DriveBackForward : DareLib/Dare/setAPI_type  g_funcname=Ecual_GpioWriteCh  g_param=EN_MCU_PIN6_RELAY_DRV  g_type=uint8  g_size=-1
      settings: AttributesFormatString=%<g_funcname>  SourceProductName=Dare Library
  DriverBackBackward : DareLib/Dare/setAPI_type  g_funcname=Ecual_GpioWriteCh  g_param=EN_MCU_PIN7_RELAY_DRV  g_type=uint8  g_size=-1
      settings: AttributesFormatString=%<g_funcname>  SourceProductName=Dare Library
  DriverFrontDown : DareLib/Dare/setAPI_type  g_funcname=Ecual_GpioWriteCh  g_param=EN_MCU_PIN4_RELAY_DRV  g_type=uint8  g_size=-1
      settings: AttributesFormatString=%<g_funcname>  SourceProductName=Dare Library
  DriverFrontUp : DareLib/Dare/setAPI_type  g_funcname=Ecual_GpioWriteCh  g_param=EN_MCU_PIN9_RELAY_DRV  g_type=uint8  g_size=-1
      settings: AttributesFormatString=%<g_funcname>  SourceProductName=Dare Library
  DriverHeightDown : DareLib/Dare/setAPI_type  g_funcname=Ecual_GpioWriteCh  g_param=EN_MCU_PIN1_RELAY_DRV  g_type=uint8  g_size=-1
      settings: AttributesFormatString=%<g_funcname>  SourceProductName=Dare Library
  DriverHeightUp : DareLib/Dare/setAPI_type  g_funcname=Ecual_GpioWriteCh  g_param=EN_MCU_PIN2_RELAY_DRV  g_type=uint8  g_size=-1
      settings: AttributesFormatString=%<g_funcname>  SourceProductName=Dare Library
  DriverLengthBackward : DareLib/Dare/setAPI_type  g_funcname=Ecual_GpioWriteCh  g_param=EN_MCU_PIN8_RELAY_DRV  g_type=uint8  g_size=-1
      settings: AttributesFormatString=%<g_funcname>  SourceProductName=Dare Library
  DriverLengthForward : DareLib/Dare/setAPI_type  g_funcname=Ecual_GpioWriteCh  g_param=EN_MCU_PIN3_RELAY_DRV  g_type=uint8  g_size=-1
      settings: AttributesFormatString=%<g_funcname>  SourceProductName=Dare Library
  wires:
  Height/1 -> Bus Selector/1
  Bus Selector/1 -> DriverHeightUp/1  "<Up_Forward>"
  Bus Selector/2 -> DriverHeightDown/1  "<Down_Backward>"
  Length/1 -> Bus Selector1/1
  Bus Selector1/1 -> DriverLengthBackward/1  "<Up_Forward>"
  Bus Selector1/2 -> DriverLengthForward/1  "<Down_Backward>"
  Back/1 -> Bus Selector2/1
  Bus Selector2/1 -> DriveBackForward/1  "<Up_Forward>"
  Bus Selector2/2 -> DriverBackBackward/1  "<Down_Backward>"
  Front/1 -> Bus Selector3/1
  Bus Selector3/1 -> DriverFrontUp/1  "<Up_Forward>"
  Bus Selector3/2 -> DriverFrontDown/1  "<Down_Backward>"

== system Appl_PaAdjustModel/LogicCtrl/LocalAdjustCtrl/AdjustRequestPriority ==
  InputSignalBus : Inport
  Bus Selector3 : BusSelector  OutputSignals=HarSwitchCmd.PaMtr_HeightSwitchCmd,HarSwitchCmd.PaMtr_LengthSwitchCmd,HarSwitchCmd.PaMtr_BackSwitchCmd,HarSwitchCmd.PaMtr_FrontSwitchCmd,MemoryReq.PaMtr_MemoryHeightReqPosi,MemoryReq.PaMtr_MemoryLengthReqPosi,MemoryReq.PaMtr_MemoryBackReqPosi,MemoryReq.PaMtr_MemoryFrontReqPosi,WelcomeReq.PaMtr_WelcomeLengthReqPosi,WelcomeReq.PaMtr_WelcomeBackReqPosi,LearnReq.PaMtr_HeightLearnCmd,LearnReq.PaMtr_LengthLearnCmd,LearnReq.PaMtr_BackLearnCmd,LearnReq.PaMtr_FrontLearnCmd,ResetReq.PaMtr_ResetHeightReqPosi,ResetReq.PaMtr_ResetLengthReqPosi,ResetReq.PaMtr_ResetBackReqPosi,ResetReq.PaMtr_ResetFrontReqPosi
  PaMotorAdjustmentPriorityProcessing : Stateflow chart  TreatAsAtomicUnit=on
  setAPI_type : DareLib/Dare/setAPI_type  Commented=on  g_funcname=Srvl_Set_D_SimuIndex_TestValue2  g_param=D_SimuIndex_TestValue2  g_type=uint8  g_size=-1
      settings: AttributesFormatString=%<g_funcname>  SourceProductName=Dare Library
  MotorActType : Outport
  SeatHeightPosiReq : Outport  Port=2
  SeatLengthPosiReq : Outport  Port=3
  SeatBackPosiReq : Outport  Port=4
  SeatFrontPosiReq : Outport  Port=5
  HeightManualAdjSw : Outport  Port=6
  LengthManualAdjSw : Outport  Port=7
  BackManualAdjSw : Outport  Port=8
  FrontManualAdjSw : Outport  Port=9
  wires:
  PaMotorAdjustmentPriorityProcessing/1(MotorActionType) -> MotorActType/1
  PaMotorAdjustmentPriorityProcessing/2(SeatHeightPosiReq) -> SeatHeightPosiReq/1
  PaMotorAdjustmentPriorityProcessing/3(SeatLengthPosiReq) -> SeatLengthPosiReq/1
  PaMotorAdjustmentPriorityProcessing/4(SeatBackPosiReq) -> SeatBackPosiReq/1
  PaMotorAdjustmentPriorityProcessing/5(SeatFrontPosiReq) -> SeatFrontPosiReq/1
  PaMotorAdjustmentPriorityProcessing/6(HeightManualAdjSw) -> HeightManualAdjSw/1
  PaMotorAdjustmentPriorityProcessing/7(LengthManualAdjSw) -> LengthManualAdjSw/1
  PaMotorAdjustmentPriorityProcessing/8(BackManualAdjSw) -> BackManualAdjSw/1
  PaMotorAdjustmentPriorityProcessing/9(FrontManualAdjSw) -> FrontManualAdjSw/1
  PaMotorAdjustmentPriorityProcessing/10(TestValue2) -> setAPI_type/1
  InputSignalBus/1 -> Bus Selector3/1
  Bus Selector3/1 -> PaMotorAdjustmentPriorityProcessing/1(PaMtr_HeightSwitchCmd)  "<PaMtr_HeightSwitchCmd>"
  Bus Selector3/2 -> PaMotorAdjustmentPriorityProcessing/2(PaMtr_LengthSwitchCmd)  "<PaMtr_LengthSwitchCmd>"
  Bus Selector3/3 -> PaMotorAdjustmentPriorityProcessing/3(PaMtr_BackSwitchCmd)  "<PaMtr_BackSwitchCmd>"
  Bus Selector3/4 -> PaMotorAdjustmentPriorityProcessing/4(PaMtr_FrontSwitchCmd)  "<PaMtr_FrontSwitchCmd>"
  Bus Selector3/5 -> PaMotorAdjustmentPriorityProcessing/5(PaMtr_MemoryHeightReqPosi)  "<PaMtr_MemoryHeightReqPosi>"
  Bus Selector3/6 -> PaMotorAdjustmentPriorityProcessing/6(PaMtr_MemoryLengthReqPosi)  "<PaMtr_MemoryLengthReqPosi>"
  Bus Selector3/7 -> PaMotorAdjustmentPriorityProcessing/7(PaMtr_MemoryBackReqPosi)  "<PaMtr_MemoryBackReqPosi>"
  Bus Selector3/8 -> PaMotorAdjustmentPriorityProcessing/8(PaMtr_MemoryFrontReqPosi)  "<PaMtr_MemoryFrontReqPosi>"
  Bus Selector3/9 -> PaMotorAdjustmentPriorityProcessing/9(PaMtr_WelcomeLengthReqPosi)  "<PaMtr_WelcomeLengthReqPosi>"
  Bus Selector3/10 -> PaMotorAdjustmentPriorityProcessing/10(PaMtr_WelcomeBackReqPosi)  "<PaMtr_WelcomeBackReqPosi>"
  Bus Selector3/11 -> PaMotorAdjustmentPriorityProcessing/11(PaMtr_HeightLearnCmd)  "<PaMtr_HeightLearnCmd>"
  Bus Selector3/12 -> PaMotorAdjustmentPriorityProcessing/12(PaMtr_LengthLearnCmd)  "<PaMtr_LengthLearnCmd>"
  Bus Selector3/13 -> PaMotorAdjustmentPriorityProcessing/13(PaMtr_BackLearnCmd)  "<PaMtr_BackLearnCmd>"
  Bus Selector3/14 -> PaMotorAdjustmentPriorityProcessing/14(PaMtr_FrontLearnCmd)  "<PaMtr_FrontLearnCmd>"
  Bus Selector3/15 -> PaMotorAdjustmentPriorityProcessing/15(PaMtr_ResetHeightReqPosi)  "<PaMtr_ResetHeightReqPosi>"
  Bus Selector3/16 -> PaMotorAdjustmentPriorityProcessing/16(PaMtr_ResetLengthReqPosi)  "<PaMtr_ResetLengthReqPosi>"
  Bus Selector3/17 -> PaMotorAdjustmentPriorityProcessing/17(PaMtr_ResetBackReqPosi)  "<PaMtr_ResetBackReqPosi>"
  Bus Selector3/18 -> PaMotorAdjustmentPriorityProcessing/18(PaMtr_ResetFrontReqPosi)  "<PaMtr_ResetFrontReqPosi>"

== system Appl_PaAdjustModel/LogicCtrl/LocalAdjustCtrl/CrankAndVoltageDeal ==
  CrankAndVoltageDealInput : Inport
  Bus Creator : BusCreator  Inputs=4
  Bus Selector9 : BusSelector  OutputSignals=RteInputBus.Power.PaMtr_PowerModeStatus,RteInputBus.Power.PaMtr_VoltMode,SeatMoveCmd.H_SeatMoveCmd,SeatMoveCmd.L_SeatMoveCmd,SeatMoveCmd.B_SeatMoveCmd,SeatMoveCmd.F_SeatMoveCmd,OTABanFlag,RteInputBus.Power.PaMtr_VoltSatisfy
  CrankUnloading : Stateflow chart  TreatAsAtomicUnit=on
  MotorCmd : Outport
  wires:
  CrankAndVoltageDealInput/1 -> Bus Selector9/1
  Bus Selector9/1 -> CrankUnloading/1(PowerMode)  "<PaMtr_PowerModeStatus>"
  Bus Selector9/2 -> CrankUnloading/2(MtrCtrl_VoltMode)  "<PaMtr_VoltMode>"
  Bus Selector9/3 -> CrankUnloading/3(HeightMotorDirection)  "<H_SeatMoveCmd>"
  Bus Selector9/4 -> CrankUnloading/4(LengthMotorDirection)  "<L_SeatMoveCmd>"
  Bus Selector9/7 -> CrankUnloading/7(DrAdj_OTABanFlag)  "<OTABanFlag>"
  Bus Selector9/8 -> CrankUnloading/8(MtrCtrl_VoltSatisfy)  "<PaMtr_VoltSatisfy>"
  Bus Creator/1 -> MotorCmd/1
  CrankUnloading/1(HeightMotorCmd) -> Bus Creator/1
  CrankUnloading/2(LengthMotorCmd) -> Bus Creator/2
  CrankUnloading/3(BackMotorCmd) -> Bus Creator/3
  CrankUnloading/4(FrontMotorCmd) -> Bus Creator/4
  Bus Selector9/5 -> CrankUnloading/5(BackMotorDirection)  "<B_SeatMoveCmd>"
  Bus Selector9/6 -> CrankUnloading/6(FrontMotorDirection)  "<F_SeatMoveCmd>"

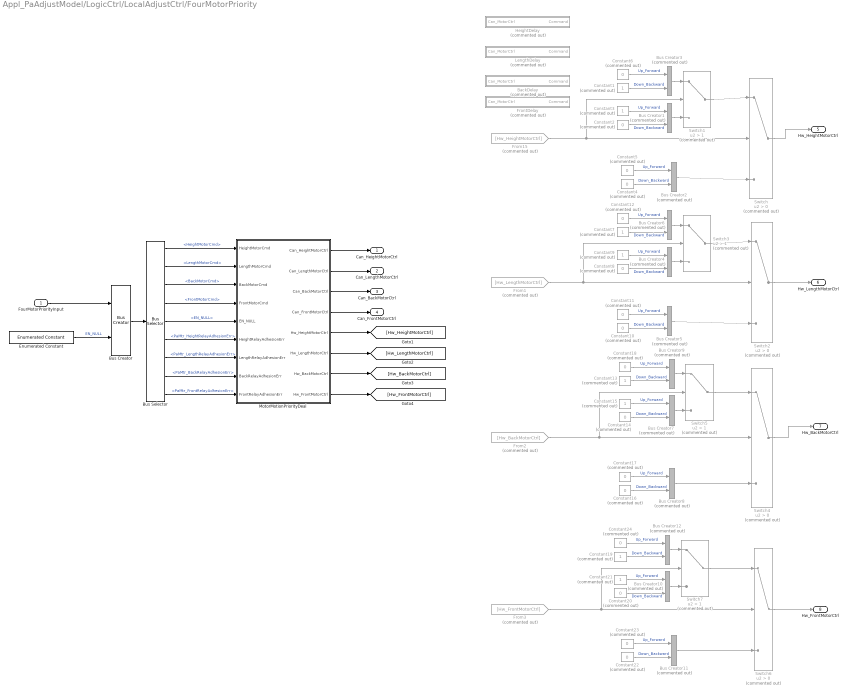
== system Appl_PaAdjustModel/LogicCtrl/LocalAdjustCtrl/FourMotorPriority ==
  FourMotorPriorityInput : Inport
  BackDelay : Stateflow chart  Commented=on  TreatAsAtomicUnit=on
  Bus Creator : BusCreator  Inputs=2
  Bus Creator{1..12} (12 alike) : BusCreator  Commented=on  Inputs=2
  Bus Selector : BusSelector  OutputSignals=FourMotorPriorityInput.MotorCmd.HeightMotorCmd,FourMotorPriorityInput.MotorCmd.LengthMotorCmd,FourMotorPriorityInput.MotorCmd.BackMotorCmd,FourMotorPriorityInput.MotorCmd.FrontMotorCmd,EN_NULL,FourMotorPriorityInput.RteInputBus.ErrSts.PaMtr_HeightRelayAdhesionErr,FourMotorPriorityInput.RteInputBus.ErrSts.PaMtr_LengthRelayAdhesionErr,FourMotorPriorityInput.RteInputBus.ErrSts.PaMtr_BackRelayAdhesionErr,FourMotorPriorityInput.RteInputBus.ErrSts.PaMtr_FrontRelayAdhesionErr
  Constant{1,3,7,9,13,15,19,21} (8 alike) : Constant  Commented=on  OutDataTypeStr=uint8
  Constant{2,4..6,8,10..12,14,16..18,20,22..24} (16 alike) : Constant  Commented=on  Value=0  OutDataTypeStr=uint8
  Enumerated Constant : simulink/Sources/Enumerated Constant  OutDataTypeStr=Enum: enSeatMoveCmd  Value=enSeatMoveCmd.EN_NULL  SampleTime=inf
      settings: SourceProductName=Simulink
  From1 : From  Commented=on  GotoTag=Hw_LengthMotorCtrl
  From15 : From  Commented=on  GotoTag=Hw_HeightMotorCtrl
  From2 : From  Commented=on  GotoTag=Hw_BackMotorCtrl
  From3 : From  Commented=on  GotoTag=Hw_FrontMotorCtrl
  FrontDelay : Stateflow chart  Commented=on  TreatAsAtomicUnit=on
  HeightDelay : Stateflow chart  Commented=on  TreatAsAtomicUnit=on
  LengthDelay : Stateflow chart  Commented=on  TreatAsAtomicUnit=on
  MotorMotionPriorityDeal : Stateflow chart  TreatAsAtomicUnit=on
  Switch{,2,4,6} (4 alike) : Switch  Commented=on  Criteria=u2 > Threshold
  Switch{1,3,5,7} (4 alike) : Switch  Commented=on  Criteria=u2 > Threshold  Threshold=1
  Can_HeightMotorCtrl : Outport
  Can_LengthMotorCtrl : Outport  Port=2
  Can_BackMotorCtrl : Outport  Port=3
  Can_FrontMotorCtrl : Outport  Port=4
  Hw_HeightMotorCtrl : Outport  Port=5
  Hw_LengthMotorCtrl : Outport  Port=6
  Hw_BackMotorCtrl : Outport  Port=7
  Hw_FrontMotorCtrl : Outport  Port=8
  wires:
  Switch1/1 -> Switch/1
  Bus Creator2/1 -> Switch/3
  Switch/1 -> Hw_HeightMotorCtrl/1
  Constant3/1 -> Bus Creator1/1  "Up_Forward"
  Constant2/1 -> Bus Creator1/2  "Down_Backward"
  Bus Creator1/1 -> Switch1/3
  Constant4/1 -> Bus Creator2/2  "Down_Backward"
  Constant5/1 -> Bus Creator2/1  "Up_Forward"
  Constant1/1 -> Bus Creator3/2  "Down_Backward"
  Constant6/1 -> Bus Creator3/1  "Up_Forward"
  Bus Creator3/1 -> Switch1/1
  Bus Creator5/1 -> Switch2/3
  Constant7/1 -> Bus Creator6/2  "Down_Backward"
  Bus Creator6/1 -> Switch3/1
  Constant10/1 -> Bus Creator5/2  "Down_Backward"
  Constant11/1 -> Bus Creator5/1  "Up_Forward"
  Bus Creator4/1 -> Switch3/3
  Switch3/1 -> Switch2/1
  Constant8/1 -> Bus Creator4/2  "Down_Backward"
  Constant12/1 -> Bus Creator6/1  "Up_Forward"
  Constant9/1 -> Bus Creator4/1  "Up_Forward"
  Switch2/1 -> Hw_LengthMotorCtrl/1
  Bus Creator8/1 -> Switch4/3
  Constant13/1 -> Bus Creator9/2  "Down_Backward"
  Bus Creator9/1 -> Switch5/1
  Constant16/1 -> Bus Creator8/2  "Down_Backward"
  Constant17/1 -> Bus Creator8/1  "Up_Forward"
  Bus Creator7/1 -> Switch5/3
  Switch5/1 -> Switch4/1
  Constant14/1 -> Bus Creator7/2  "Down_Backward"
  Constant18/1 -> Bus Creator9/1  "Up_Forward"
  Constant15/1 -> Bus Creator7/1  "Up_Forward"
  Bus Creator11/1 -> Switch6/3
  Constant19/1 -> Bus Creator12/2  "Down_Backward"
  Bus Creator12/1 -> Switch7/1
  Constant22/1 -> Bus Creator11/2  "Down_Backward"
  Constant23/1 -> Bus Creator11/1  "Up_Forward"
  Bus Creator10/1 -> Switch7/3
  Switch7/1 -> Switch6/1
  Constant20/1 -> Bus Creator10/2  "Down_Backward"
  Constant24/1 -> Bus Creator12/1  "Up_Forward"
  Constant21/1 -> Bus Creator10/1  "Up_Forward"
  Switch4/1 -> Hw_BackMotorCtrl/1
  Switch6/1 -> Hw_FrontMotorCtrl/1
  MotorMotionPriorityDeal/5(Hw_HeightMotorCtrl) -> [Hw_HeightMotorCtrl]
  From15/1 -> Switch1/2, Switch/2
  MotorMotionPriorityDeal/6(Hw_LengthMotorCtrl) -> [Hw_LengthMotorCtrl]
  From1/1 -> Switch3/2, Switch2/2
  MotorMotionPriorityDeal/7(Hw_BackMotorCtrl) -> [Hw_BackMotorCtrl]
  From2/1 -> Switch5/2, Switch4/2
  MotorMotionPriorityDeal/8(Hw_FrontMotorCtrl) -> [Hw_FrontMotorCtrl]
  From3/1 -> Switch7/2, Switch6/2
  FourMotorPriorityInput/1 -> Bus Creator/1
  Enumerated Constant/1 -> Bus Creator/2  "EN_NULL"
  Bus Creator/1 -> Bus Selector/1
  MotorMotionPriorityDeal/1(Can_HeightMotorCtrl) -> Can_HeightMotorCtrl/1
  MotorMotionPriorityDeal/2(Can_LengthMotorCtrl) -> Can_LengthMotorCtrl/1
  MotorMotionPriorityDeal/3(Can_BackMotorCtrl) -> Can_BackMotorCtrl/1
  MotorMotionPriorityDeal/4(Can_FrontMotorCtrl) -> Can_FrontMotorCtrl/1
  Bus Selector/1 -> MotorMotionPriorityDeal/1(HeightMotorCmd)  "<HeightMotorCmd>"
  Bus Selector/2 -> MotorMotionPriorityDeal/2(LengthMotorCmd)  "<LengthMotorCmd>"
  Bus Selector/3 -> MotorMotionPriorityDeal/3(BackMotorCmd)  "<BackMotorCmd>"
  Bus Selector/4 -> MotorMotionPriorityDeal/4(FrontMotorCmd)  "<FrontMotorCmd>"
  Bus Selector/5 -> MotorMotionPriorityDeal/5(EN_NULL)  "<EN_NULL>"
  Bus Selector/6 -> MotorMotionPriorityDeal/6(HeightRelayAdhesionErr)  "<PaMtr_HeightRelayAdhesionErr>"
  Bus Selector/7 -> MotorMotionPriorityDeal/7(LengthRelayAdhesionErr)  "<PaMtr_LengthRelayAdhesionErr>"
  Bus Selector/8 -> MotorMotionPriorityDeal/8(BackRelayAdhesionErr)  "<PaMtr_BackRelayAdhesionErr>"
  Bus Selector/9 -> MotorMotionPriorityDeal/9(FrontRelayAdhesionErr)  "<PaMtr_FrontRelayAdhesionErr>"
